simulink library "motohawk_control_primitives_motoshare_lib"  (Simulink 6.3)
undefined symbols (not defined in the file or in its folder): motohawk_vardec_config_group, motohawk_vardec_path, p, samp_time, SampleTime
libraries: MotoHawk_lib x76, motohawk_control_primitives_lib x30, simulink x9
(part 2 of 3)

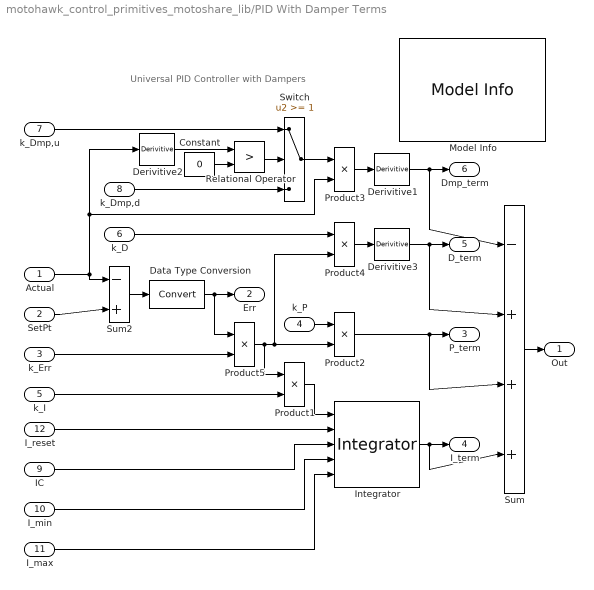
== system motohawk_control_primitives_motoshare_lib/PID With Damper Terms ==
  note: Universal PID Controller
      | with Dampers
  Actual : Inport
  SetPt : Inport  Port=2
  k_Err : Inport  Port=3
  k_P : Inport  Port=4
  k_I : Inport  Port=5
  k_D : Inport  Port=6
  k_Dmp,u : Inport  Port=7
  k_Dmp,d : Inport  Port=8
  IC : Inport  Port=9
  I_min : Inport  Port=10
  I_max : Inport  Port=11
  I_reset : Inport  Port=12
  Constant : Constant  Value=0
  Data Type Conversion : DataTypeConversion  SaturateOnIntegerOverflow=on  RndMeth=Zero
  Derivitive1 : motohawk_control_primitives_lib/Derivitive  samp_time=samp_time
  Derivitive2 : motohawk_control_primitives_lib/Derivitive  samp_time=samp_time
  Derivitive3 : motohawk_control_primitives_lib/Derivitive  samp_time=samp_time
  Integrator : motohawk_control_primitives_lib/Integrator  samp_time=samp_time
  Model Info : simulink/Model-Wide Utilities/Model Info  InitialBlockCM=None  BlockCM=None  Frame=on  DisplayStringWithTags=|  HorizontalTextAlignment=Center  LeftAlignmentValue=0.5  SourceBlockDiagram=motohawk_control_primitives_lib  TagMaxNumber=20
      | Model Info:
      | Author: Suhre, Poorman
      | %<Created>
      | %<ModifiedDate>
      | Version: %<ModelVersion>
      | MotoTron Confidential
      | and Propietary
  Product{1..5} (5 alike) : Product  InputSameDT=on
  Relational Operator : RelationalOperator  Operator=>  ZeroCross=off  InputSameDT=on
  Sum : Sum  Inputs=-|+|+|+  SaturateOnIntegerOverflow=on  InputSameDT=on
  Sum2 : Sum  Inputs=-|+  SaturateOnIntegerOverflow=on  InputSameDT=on
  Switch : Switch  Threshold=1  ZeroCross=off  InputSameDT=on
  Out : Outport
  Err : Outport  Port=2
  P_term : Outport  Port=3
  I_term : Outport  Port=4
  D_term : Outport  Port=5
  Dmp_term : Outport  Port=6
  wires:
  Product3/1 -> Derivitive1/1
  k_Dmp,u/1 -> Switch/1
  k_Dmp,d/1 -> Switch/3
  Switch/1 -> Product3/1
  Derivitive2/1 -> Relational Operator/1
  Relational Operator/1 -> Switch/2
  Constant/1 -> Relational Operator/2
  I_max/1 -> Integrator/5
  I_min/1 -> Integrator/4
  Data Type Conversion/1 -> Product5/1, Err/1
  k_Err/1 -> Product5/2
  I_reset/1 -> Integrator/2
  Actual/1 -> Sum2/1, Derivitive2/1, Product3/2
  k_P/1 -> Product2/1
  k_I/1 -> Product1/2
  Product1/1 -> Integrator/1
  Product2/1 -> P_term/1, Sum/3
  Integrator/1 -> I_term/1, Sum/4
  Sum/1 -> Out/1
  IC/1 -> Integrator/3
  Product5/1 -> Product1/1, Product2/2, Product4/2
  Sum2/1 -> Data Type Conversion/1
  SetPt/1 -> Sum2/2
  k_D/1 -> Product4/1
  Product4/1 -> Derivitive3/1
  Derivitive3/1 -> D_term/1, Sum/2
  Derivitive1/1 -> Dmp_term/1, Sum/1

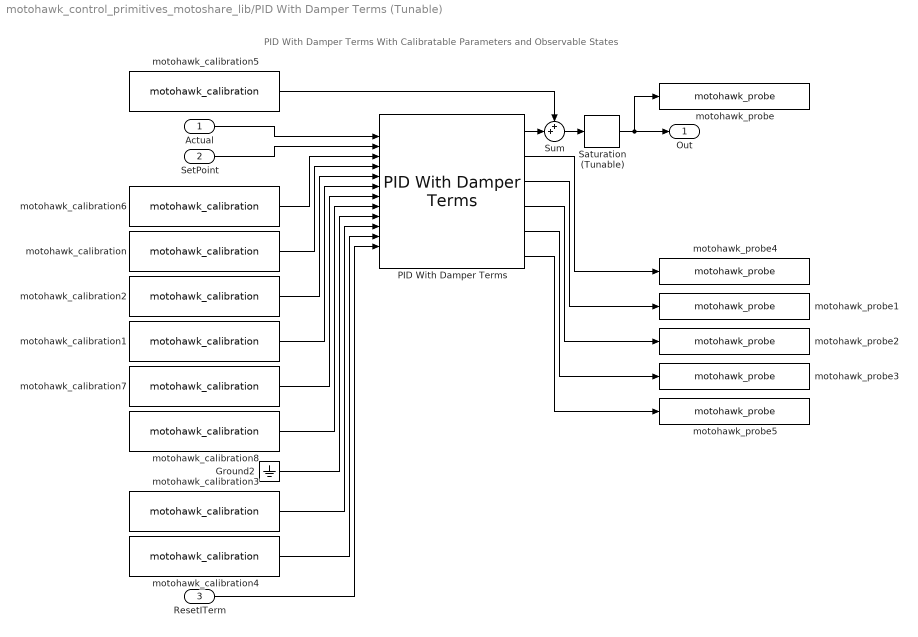
== system motohawk_control_primitives_motoshare_lib/PID With Damper Terms (Tunable) ==
  note: PID With Damper Terms
      | With Calibratable Parameters and Observable States
  Actual : Inport
  SetPoint : Inport  Port=2
  ResetITerm : Inport  Port=3
  Ground2 : Ground
  PID With Damper Terms : motohawk_control_primitives_lib/PID With Damper Terms  Description=|  samp_time=SampleTime
      | /* Name: ErrorGain Unit:mult ClassID:VAR StorageID:FLASH Access:RW4+RW3+NA2+NA1 TypeID:UINT4                   
      |    Gain:0.000000001 Min:0.000000000 Max:4.000000000 Format:10.9 UpdateID:REMOTE Help:"This gain is applied to "
      |    "the error term before it is used to calculate the P, I and D terms." VardecSig:6C */                       
      |                                                                                                                
      | /* Name: ITermLowerLim Unit:0 ClassID:VAR StorageID:FLASH Access:RW4+RW3+NA2+NA1 TypeID:SINT2 Gain:0.1         
      |    Min:-3276.8 Max:3276.7 Format:5.1 UpdateID:REMOTE Help:"Lower limit on the I-term value." VardecSig:6C */   
      |                                                                                                                
      | /* Name: ITermUpperLim ClassID:VAR StorageID:FLASH Access:RW4+RW3+NA2+NA1 TypeID:SINT2 Gain:0.1 Min:-3276.8    
      |    Max:3276.7 Format:5.1 UpdateID:REMOTE Help:"Upper limit on I-term value." VardecSig:6C */                   
      |                                                                                                                
      | /* Name: PIDOutLowerLim ClassID:VAR StorageID:FLASH Access:RW4+RW3+NA2+NA1 TypeID:SINT2 Gain:0.1               
      |    Min:-3276.8 Max:3276.7 Format:5.1 UpdateID:REMOTE Help:"Lower limit on PID output." VardecSig:6C */         
      |                                                                                                                
      | /* Name: PIDOutUpperLim ClassID:VAR StorageID:FLASH Access:RW4+RW3+NA2+NA1 TypeID:SINT2 Gain:0.1               
      |    Min:-3276.8 Max:3276.7 Format:3.1 UpdateID:REMOTE Help:"Upper limit on PID output." VardecSig:6C */         
      |                                                                                                                
      | /* Name: PIDError ClassID:VAR StorageID:RAM Access:RO4+RO3+NA2+NA1 TypeID:SINT2 Gain:1 Min:-32768.00           
      |    Max:32767.00 Format:4.2 UpdateID:BACKGND Help:"Current controller error input value." VardecSig:6C */       
      |                                                                                                                
      | /* Name: PTerm ClassID:VAR StorageID:RAM Access:RO4+RO3+NA2+NA1 TypeID:SINT2 Gain:1 Min:-32768.00              
      |    Max:32767.00 Format:4.2 UpdateID:BACKGND Help:"Current P-term value" VardecSig:6C */                        
      |                                                                                                                
      | /* Name: ITerm ClassID:VAR StorageID:RAM Access:RO4+RO3+NA2+NA1 TypeID:SINT2 Gain:1 Min:-32768.00              
      |    Max:32767.00 Format:4.2 UpdateID:BACKGND Help:"Current I-term value" VardecSig:6C */                        
      |                                                                                                                
      | /* Name: DTerm ClassID:VAR StorageID:RAM Access:RO4+RO3+NA2+NA1 TypeID:SINT2 Gain:1 Min:-32768.00              
      |    Max:32767.00 Format:4.2 UpdateID:BACKGND Help:"Current D-term value" VardecSig:6C */                        
      |                                                                                                                
      | /* Name: DamperTerm ClassID:VAR StorageID:RAM Access:RO4+RO3+NA2+NA1 TypeID:SINT2 Gain:1 Min:-32768.00         
      |    Max:32767.00 Format:4.2 UpdateID:BACKGND Help:"Current Damper-term value" VardecSig:6C */                   
      |                                                                                                                
      | /* Name: PIDOutput ClassID:VAR StorageID:FLASH Access:RW4+RW3+NA2+NA1 TypeID:SINT2 Gain:1 Min:-32768.00        
      |    Max:32767.00 Format:4.2 UpdateID:REMOTE Help:"PID current output." VardecSig:6C */
  Saturation (Tunable) : motohawk_control_primitives_lib/Saturation (Tunable)  prefix=prefix  units=units  grp=grp
  Sum : Sum  Inputs=++|  InputSameDT=on
  motohawk_calibration : MotoHawk_lib/Calibration & Probing Blocks/motohawk_calibration  nam=[prefix 'PGain']  val=1  storage=Calibration  show_more=on  name_source=Use Parameter  data_type=Inherit from 'Default Value'  read_level=1  write_level=1  ovr_cals=on  view_as=Number  enum_struct={'Disabled', 'Enabled'}  vector_style=Wide Row  use_help_units=on  help='PID Proportional Gain'  units='mult'  use_header_enum=off  row_header_enum={}  col_header_enum={}  use_min_max=off  min_val=-inf  max_val=inf  use_precision=off  precision=''  gain=1  offset=0  exp=1  use_mototune_group=on  mototune_group=grp
  motohawk_calibration1 : MotoHawk_lib/Calibration & Probing Blocks/motohawk_calibration  nam=[prefix 'DGain']  val=1  storage=Calibration  show_more=on  name_source=Use Parameter  data_type=Inherit from 'Default Value'  read_level=1  write_level=1  ovr_cals=on  view_as=Number  enum_struct={'Disabled', 'Enabled'}  vector_style=Wide Row  use_help_units=on  help='PID Derivative Gain'  units='mult'  use_header_enum=off  row_header_enum={}  col_header_enum={}  use_min_max=off  min_val=-inf  max_val=inf  use_precision=off  precision=''  gain=1  offset=0  exp=1  use_mototune_group=on  mototune_group=grp
  motohawk_calibration2 : MotoHawk_lib/Calibration & Probing Blocks/motohawk_calibration  nam=[prefix 'IGain']  val=1  storage=Calibration  show_more=on  name_source=Use Parameter  data_type=Inherit from 'Default Value'  read_level=1  write_level=1  ovr_cals=on  view_as=Number  enum_struct={'Disabled', 'Enabled'}  vector_style=Wide Row  use_help_units=on  help='PID Integral Gain'  units='mult'  use_header_enum=off  row_header_enum={}  col_header_enum={}  use_min_max=off  min_val=-inf  max_val=inf  use_precision=off  precision=''  gain=1  offset=0  exp=1  use_mototune_group=on  mototune_group=grp
  motohawk_calibration3 : MotoHawk_lib/Calibration & Probing Blocks/motohawk_calibration  nam=[prefix 'IMin']  val=0  storage=Calibration  show_more=on  name_source=Use Parameter  data_type=Inherit from 'Default Value'  read_level=1  write_level=1  ovr_cals=on  view_as=Number  enum_struct={'Disabled', 'Enabled'}  vector_style=Wide Row  use_help_units=on  help='PID Integrator Lower Limit'  units=units  use_header_enum=off  row_header_enum={}  col_header_enum={}  use_min_max=off  min_val=-inf  max_val=inf  use_precision=off  precision=''  gain=1  offset=0  exp=1  use_mototune_group=on  mototune_group=grp
  motohawk_calibration4 : MotoHawk_lib/Calibration & Probing Blocks/motohawk_calibration  nam=[prefix 'IMax']  val=1  storage=Calibration  show_more=on  name_source=Use Parameter  data_type=Inherit from 'Default Value'  read_level=1  write_level=1  ovr_cals=on  view_as=Number  enum_struct={'Disabled', 'Enabled'}  vector_style=Wide Row  use_help_units=on  help='PID Integrator Upper Limit'  units=units  use_header_enum=off  row_header_enum={}  col_header_enum={}  use_min_max=off  min_val=-inf  max_val=inf  use_precision=off  precision=''  gain=1  offset=0  exp=1  use_mototune_group=on  mototune_group=grp
  motohawk_calibration5 : MotoHawk_lib/Calibration & Probing Blocks/motohawk_calibration  nam=[prefix 'DCOffset']  val=0  storage=Calibration  show_more=on  name_source=Use Parameter  data_type=Inherit from 'Default Value'  read_level=1  write_level=1  ovr_cals=on  view_as=Number  enum_struct={'Disabled', 'Enabled'}  vector_style=Wide Row  use_help_units=on  help='PID Output DC Offset'  units=units  use_header_enum=off  row_header_enum={}  col_header_enum={}  use_min_max=off  min_val=-inf  max_val=inf  use_precision=off  precision=''  gain=1  offset=0  exp=1  use_mototune_group=on  mototune_group=grp
  motohawk_calibration6 : MotoHawk_lib/Calibration & Probing Blocks/motohawk_calibration  nam=[prefix 'ErrorGain']  val=1  storage=Calibration  show_more=on  name_source=Use Parameter  data_type=Inherit from 'Default Value'  read_level=1  write_level=1  ovr_cals=on  view_as=Number  enum_struct={'Disabled', 'Enabled'}  vector_style=Wide Row  use_help_units=on  help='PID Error Gain'  units='mult'  use_header_enum=off  row_header_enum={}  col_header_enum={}  use_min_max=off  min_val=-inf  max_val=inf  use_precision=off  precision=''  gain=1  offset=0  exp=1  use_mototune_group=on  mototune_group=grp
  motohawk_calibration7 : MotoHawk_lib/Calibration & Probing Blocks/motohawk_calibration  nam=[prefix 'DampGainUp']  val=1  storage=Calibration  show_more=on  name_source=Use Parameter  data_type=Inherit from 'Default Value'  read_level=1  write_level=1  ovr_cals=on  view_as=Number  enum_struct={'Disabled', 'Enabled'}  vector_style=Wide Row  use_help_units=on  help='PID Damper Gain - Up Direction'  units='mult'  use_header_enum=off  row_header_enum={}  col_header_enum={}  use_min_max=off  min_val=-inf  max_val=inf  use_precision=off  precision=''  gain=1  offset=0  exp=1  use_mototune_group=on  mototune_group=grp
  motohawk_calibration8 : MotoHawk_lib/Calibration & Probing Blocks/motohawk_calibration  nam=[prefix 'DampGainDown']  val=1  storage=Calibration  show_more=on  name_source=Use Parameter  data_type=Inherit from 'Default Value'  read_level=1  write_level=1  ovr_cals=on  view_as=Number  enum_struct={'Disabled', 'Enabled'}  vector_style=Wide Row  use_help_units=on  help='PID Damper Gain - Down Direction'  units='mult'  use_header_enum=off  row_header_enum={}  col_header_enum={}  use_min_max=off  min_val=-inf  max_val=inf  use_precision=off  precision=''  gain=1  offset=0  exp=1  use_mototune_group=on  mototune_group=grp
  motohawk_probe : MotoHawk_lib/Calibration & Probing Blocks/motohawk_probe  nam=[prefix 'Out']  show_more=on  name_source=Use Parameter  read_level=1  view_as=Number  enum_struct={'Disabled', 'Enabled'}  vector_style=Wide Row  use_help_units=on  help='PID Final Output'  units=units  use_header_enum=off  row_header_enum={}  col_header_enum={}  use_precision=off  precision=''  gain=1  offset=0  exp=1  use_mototune_group=on  mototune_group=grp
  motohawk_probe1 : MotoHawk_lib/Calibration & Probing Blocks/motohawk_probe  nam=[prefix 'PTerm']  show_more=on  name_source=Use Parameter  read_level=1  view_as=Number  enum_struct={'Disabled', 'Enabled'}  vector_style=Wide Row  use_help_units=on  help='PID Proportional Term'  units=units  use_header_enum=off  row_header_enum={}  col_header_enum={}  use_precision=off  precision=''  gain=1  offset=0  exp=1  use_mototune_group=on  mototune_group=grp
  motohawk_probe2 : MotoHawk_lib/Calibration & Probing Blocks/motohawk_probe  nam=[prefix 'ITerm']  show_more=on  name_source=Use Parameter  read_level=1  view_as=Number  enum_struct={'Disabled', 'Enabled'}  vector_style=Wide Row  use_help_units=on  help='PID Integrator Term'  units=units  use_header_enum=off  row_header_enum={}  col_header_enum={}  use_precision=off  precision=''  gain=1  offset=0  exp=1  use_mototune_group=on  mototune_group=grp
  motohawk_probe3 : MotoHawk_lib/Calibration & Probing Blocks/motohawk_probe  nam=[prefix 'DTerm']  show_more=on  name_source=Use Parameter  read_level=1  view_as=Number  enum_struct={'Disabled', 'Enabled'}  vector_style=Wide Row  use_help_units=on  help='PID Derivative Term'  units=units  use_header_enum=off  row_header_enum={}  col_header_enum={}  use_precision=off  precision=''  gain=1  offset=0  exp=1  use_mototune_group=on  mototune_group=grp
  motohawk_probe4 : MotoHawk_lib/Calibration & Probing Blocks/motohawk_probe  nam=[prefix 'Error']  show_more=on  name_source=Use Parameter  read_level=1  view_as=Number  enum_struct={'Disabled', 'Enabled'}  vector_style=Wide Row  use_help_units=on  help='PID Error Term'  units=units  use_header_enum=off  row_header_enum={}  col_header_enum={}  use_precision=off  precision=''  gain=1  offset=0  exp=1  use_mototune_group=on  mototune_group=grp
  motohawk_probe5 : MotoHawk_lib/Calibration & Probing Blocks/motohawk_probe  nam=[prefix 'DampTerm']  show_more=on  name_source=Use Parameter  read_level=1  view_as=Number  enum_struct={'Disabled', 'Enabled'}  vector_style=Wide Row  use_help_units=on  help='PID Damper Term'  units=units  use_header_enum=off  row_header_enum={}  col_header_enum={}  use_precision=off  precision=''  gain=1  offset=0  exp=1  use_mototune_group=on  mototune_group=grp
  Out : Outport
  wires:
  motohawk_calibration5/1 -> Sum/1
  Sum/1 -> Saturation (Tunable)/1
  ResetITerm/1 -> PID With Damper Terms/12
  Ground2/1 -> PID With Damper Terms/9
  motohawk_calibration1/1 -> PID With Damper Terms/6
  motohawk_calibration2/1 -> PID With Damper Terms/5
  motohawk_calibration/1 -> PID With Damper Terms/4
  PID With Damper Terms/3 -> motohawk_probe1/1
  Actual/1 -> PID With Damper Terms/1
  SetPoint/1 -> PID With Damper Terms/2
  PID With Damper Terms/1 -> Sum/2
  motohawk_calibration6/1 -> PID With Damper Terms/3
  motohawk_calibration3/1 -> PID With Damper Terms/10
  motohawk_calibration4/1 -> PID With Damper Terms/11
  PID With Damper Terms/4 -> motohawk_probe2/1
  PID With Damper Terms/5 -> motohawk_probe3/1
  PID With Damper Terms/2 -> motohawk_probe4/1
  motohawk_calibration7/1 -> PID With Damper Terms/7
  motohawk_calibration8/1 -> PID With Damper Terms/8
  PID With Damper Terms/6 -> motohawk_probe5/1
  Saturation (Tunable)/1 -> Out/1, motohawk_probe/1

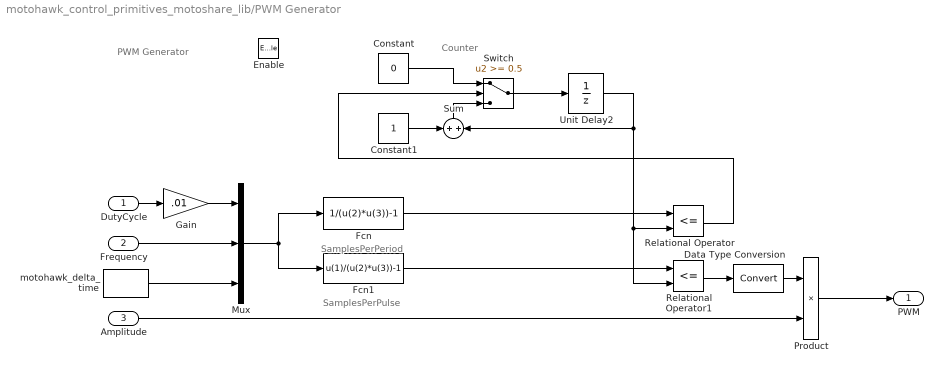
== system motohawk_control_primitives_motoshare_lib/PWM Generator ==
  note: Counter
  note: PWM Generator
  note: SamplesPerPulse
  note: SamplesPerPeriod
  DutyCycle : Inport
  Frequency : Inport  Port=2
  Amplitude : Inport  Port=3
  Enable : EnablePort  StatesWhenEnabling=reset
  Constant : Constant  Value=0
  Constant1 : Constant
  Data Type Conversion : DataTypeConversion  OutDataTypeMode=double  SaturateOnIntegerOverflow=on  RndMeth=Zero
  Fcn : Fcn  Expr=1/(u(2)*u(3))-1
  Fcn1 : Fcn  Expr=u(1)/(u(2)*u(3))-1
  Gain : Gain  Gain=.01  SaturateOnIntegerOverflow=on
  Mux : Mux  Inputs=3
  Product : Product  SaturateOnIntegerOverflow=on
  Relational Operator : RelationalOperator  Operator=<=
  Relational Operator1 : RelationalOperator  Operator=<=
  Sum : Sum  Orientation=up  SaturateOnIntegerOverflow=on  InputSameDT=on
  Switch : Switch  Threshold=0.5  SaturateOnIntegerOverflow=on  InputSameDT=on
  Unit Delay2 : UnitDelay  SampleTime=-1
  motohawk_delta_time : MotoHawk_lib/Extra Development Blocks/motohawk_delta_time  samp_time=-1  init_val=.005
  PWM : Outport  OutputWhenDisabled=reset  InitialOutput=0
  wires:
  Relational Operator/1 -> Switch/2
  Constant1/1 -> Sum/1
  Gain/1 -> Mux/1
  Data Type Conversion/1 -> Product/1
  Unit Delay2/1 -> Relational Operator1/2, Relational Operator/2, Sum/2
  Switch/1 -> Unit Delay2/1
  Constant/1 -> Switch/1
  Sum/1 -> Switch/3
  Amplitude/1 -> Product/2
  Product/1 -> PWM/1
  Relational Operator1/1 -> Data Type Conversion/1
  Fcn1/1 -> Relational Operator1/1
  Fcn/1 -> Relational Operator/1
  Mux/1 -> Fcn1/1, Fcn/1
  motohawk_delta_time/1 -> Mux/3
  Frequency/1 -> Mux/2
  DutyCycle/1 -> Gain/1

== system motohawk_control_primitives_motoshare_lib/Polynomial (Tunable) ==
  note: Evaluate polynomial using Horner's Rule.
      |      y = polyval( p, u, [], mu )
      | where
      |      p = polynomial coefficients and
      |      mu(1) = mean and
      |      mu(2) = standard deviation of fitted data.
      | See MATLAB "help polyfit" for more.
      | Note:  Degree of polynomial is fixed at compile time.
      | MotoTune can change coefficients, centering/scaling values.
  note: Evaluate Polynomial using Horner's Rule.
  u : Inport
  Constant : Constant  Value=[0 1]
  Demux : Demux  Outputs=2
  Horner's Rule : Subsystem
  Product0 : Product  Inputs=*/  SaturateOnIntegerOverflow=on
  Signal Specification0 : SignalSpecification  Dimensions=2
  Signal Specification1 : SignalSpecification  Dimensions=length(p)
  Sum : Sum  Inputs=|+-  SaturateOnIntegerOverflow=on  InputSameDT=on
  motohawk_calibration1 : MotoHawk_lib/Calibration & Probing Blocks/motohawk_calibration  nam=[prefix 'Polynomial']  val=ones(1,numcoef)  storage=Calibration  show_more=on  name_source=Use Parameter  data_type=Inherit from 'Default Value'  read_level=1  write_level=1  ovr_cals=on  view_as=Number  enum_struct={'Disabled', 'Enabled'}  vector_style=Wide Row  use_help_units=on  help='[ A_n ... A_0 ]'  units=''  use_header_enum=off  row_header_enum={}  col_header_enum={}  use_min_max=on  min_val=-inf  max_val=inf  use_precision=on  precision='1.14'  gain=1  offset=0  exp=1  use_mototune_group=on  mototune_group=grp
  y : Outport
  wires:
  Signal Specification0/1 -> Demux/1
  Signal Specification1/1 -> Horner's Rule/2(p)
  Horner's Rule/1(y) -> y/1
  motohawk_calibration1/1 -> Signal Specification1/1
  Product0/1 -> Horner's Rule/1(u_hat)
  Demux/2 -> Product0/2
  Constant/1 -> Signal Specification0/1
  Sum/1 -> Product0/1
  Demux/1 -> Sum/2
  u/1 -> Sum/1

== system motohawk_control_primitives_motoshare_lib/Rising Edge ==
  note: Detect Rising Edge of Signal
      | using Discrete Unit Delay
  In : Inport
  Data Type Conversion : DataTypeConversion  OutDataTypeMode=boolean  SaturateOnIntegerOverflow=on  RndMeth=Zero
  Logical Operator : Logic
  Logical Operator1 : Logic  Operator=NOT
  Unit Delay : UnitDelay  SampleTime=-1
  Rise : Outport
  wires:
  Data Type Conversion/1 -> Unit Delay/1, Logical Operator/1
  Logical Operator1/1 -> Logical Operator/2
  Unit Delay/1 -> Logical Operator1/1
  Logical Operator/1 -> Rise/1
  In/1 -> Data Type Conversion/1

== system motohawk_control_primitives_motoshare_lib/Saturate Divide ==
  note: When the divisor is less than the numerator,
      | saturate and output one.
  note: This is useful when dividing dT by a Time Constant.
      | It also avoids a divide by zero.
  X : Inport
  Inport : Inport  Port=2
  If : If  NumInputs=2  IfExpression=u2 < u1
  Merge : Merge
  Normal Divide : Subsystem
  Output One : Subsystem
  " " : Outport
  wires:
  X/1 -> Normal Divide/1(X), If/1
  Merge/1 -> " "/1
  Normal Divide/1(" ") -> Merge/1
  Output One/1(" ") -> Merge/2
  If/2 -> Normal Divide/Action
  If/1 -> Output One/Action
  Inport/1 -> Normal Divide/2(Inport), If/2

== system motohawk_control_primitives_motoshare_lib/Saturation ==
  note: Output 'In' when between Min and Max,
      | and saturate against limits otherwise.
  in : Inport
  min : Inport  Port=2
  max : Inport  Port=3
  MinMax : MinMax  Function=max  Inputs=2  ZeroCross=off  SaturateOnIntegerOverflow=on  InputSameDT=on
  MinMax1 : MinMax  Inputs=2  ZeroCross=off  SaturateOnIntegerOverflow=on  InputSameDT=on
  out : Outport
  wires:
  MinMax/1 -> MinMax1/1
  in/1 -> MinMax/1
  min/1 -> MinMax/2
  max/1 -> MinMax1/2
  MinMax1/1 -> out/1

== system motohawk_control_primitives_motoshare_lib/Saturation (Tunable) ==
  note: Calibratable wrapper around the Saturation block
  In : Inport
  Saturation : motohawk_control_primitives_lib/Saturation
  motohawk_calibration : MotoHawk_lib/Calibration & Probing Blocks/motohawk_calibration  nam=[prefix 'LwrLim']  val=0  storage=Calibration  show_more=on  name_source=Use Parameter  data_type=Inherit via back propagation  read_level=1  write_level=1  ovr_cals=on  view_as=Number  enum_struct={'Disabled', 'Enabled'}  vector_style=Wide Row  use_help_units=off  help='Lower Limit Value'  units=units  use_header_enum=off  row_header_enum={}  col_header_enum={}  use_min_max=on  min_val=-inf  max_val=inf  use_precision=off  precision=''  gain=1  offset=0  exp=1  use_mototune_group=on  mototune_group=grp
  motohawk_calibration1 : MotoHawk_lib/Calibration & Probing Blocks/motohawk_calibration  nam=[prefix 'UprLim']  val=1  storage=Calibration  show_more=on  name_source=Use Parameter  data_type=Inherit via back propagation  read_level=1  write_level=1  ovr_cals=on  view_as=Number  enum_struct={'Disabled', 'Enabled'}  vector_style=Wide Row  use_help_units=off  help='Upper Limit Value'  units=units  use_header_enum=off  row_header_enum={}  col_header_enum={}  use_min_max=on  min_val=-inf  max_val=inf  use_precision=off  precision=''  gain=1  offset=0  exp=1  use_mototune_group=on  mototune_group=grp
  Out : Outport
  wires:
  Saturation/1 -> Out/1
  motohawk_calibration/1 -> Saturation/2
  In/1 -> Saturation/1
  motohawk_calibration1/1 -> Saturation/3

== system motohawk_control_primitives_motoshare_lib/Simple PD ==
  note: Simple PD Controller
  Actual : Inport
  SetPt : Inport  Port=2
  k_P : Inport  Port=3
  k_D : Inport  Port=4
  Data Type Conversion1 : DataTypeConversion  SaturateOnIntegerOverflow=on  RndMeth=Zero
  Derivitive3 : motohawk_control_primitives_lib/Derivitive  samp_time=samp_time
  Model Info : simulink/Model-Wide Utilities/Model Info  InitialBlockCM=None  BlockCM=None  Frame=on  DisplayStringWithTags=|  HorizontalTextAlignment=Center  LeftAlignmentValue=0.5  SourceBlockDiagram=motohawk_control_primitives_lib  TagMaxNumber=20
      | Model Info:
      | Author: Poorman
      | %<ModifiedDate>
      | Version: %<ModelVersion>
      | MotoTron Confidential
      | and Propietary
  Product1 : Product  InputSameDT=on
  Product5 : Product  InputSameDT=on
  Sum1 : Sum  Inputs=+|+  SaturateOnIntegerOverflow=on  InputSameDT=on
  Sum2 : Sum  Inputs=-|||+  SaturateOnIntegerOverflow=on  InputSameDT=on
  Out : Outport
  wires:
  Data Type Conversion1/1 -> Product5/2, Product1/1
  Actual/1 -> Sum2/1
  k_P/1 -> Product1/2
  Sum2/1 -> Data Type Conversion1/1
  SetPt/1 -> Sum2/2
  k_D/1 -> Product5/1
  Product5/1 -> Derivitive3/1
  Sum1/1 -> Out/1
  Derivitive3/1 -> Sum1/1
  Product1/1 -> Sum1/2

== system motohawk_control_primitives_motoshare_lib/Simple PI ==
  note: Simple PI Controller
  Actual : Inport
  SetPt : Inport  Port=2
  k_P : Inport  Port=3
  k_I : Inport  Port=4
  Constant : Constant
  Constant1 : Constant  Value=-inf
  Constant2 : Constant  Value=inf
  Constant3 : Constant  Value=0
  Constant4 : Constant  Value=0
  Data Type Conversion : DataTypeConversion  SaturateOnIntegerOverflow=on  RndMeth=Zero
  Integrator : motohawk_control_primitives_lib/Integrator  samp_time=samp_time
  Model Info : simulink/Model-Wide Utilities/Model Info  InitialBlockCM=None  BlockCM=None  Frame=on  DisplayStringWithTags=|  HorizontalTextAlignment=Center  LeftAlignmentValue=0.5  SourceBlockDiagram=motohawk_control_primitives_lib  TagMaxNumber=20
      | Model Info:
      | Author: Poorman
      | %<Created>
      | %<ModifiedDate>
      | Version: %<ModelVersion>
      | MotoTron Confidential
      | and Propietary
  Product1 : Product  InputSameDT=on
  Product2 : Product  InputSameDT=on
  Product3 : Product  InputSameDT=on
  Sum : Sum  Inputs=+|+  SaturateOnIntegerOverflow=on  InputSameDT=on
  Sum2 : Sum  Inputs=-|+  SaturateOnIntegerOverflow=on  InputSameDT=on
  Out : Outport
  wires:
  Constant2/1 -> Integrator/5
  Constant1/1 -> Integrator/4
  Data Type Conversion/1 -> Product3/1
  Constant/1 -> Product3/2
  Constant4/1 -> Integrator/2
  SetPt/1 -> Sum2/2
  Actual/1 -> Sum2/1
  k_P/1 -> Product2/1
  k_I/1 -> Product1/2
  Product1/1 -> Integrator/1
  Product2/1 -> Sum/1
  Integrator/1 -> Sum/2
  Sum/1 -> Out/1
  Constant3/1 -> Integrator/3
  Product3/1 -> Product2/2, Product1/1
  Sum2/1 -> Data Type Conversion/1

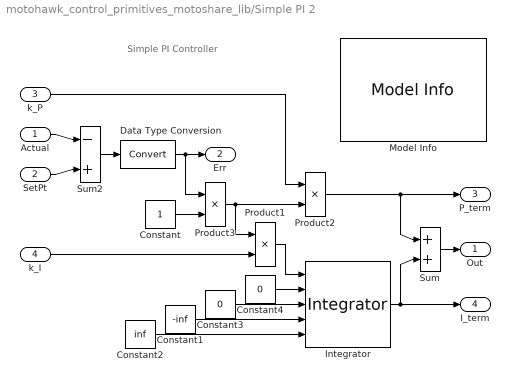
== system motohawk_control_primitives_motoshare_lib/Simple PI 2 ==
  note: Simple PI Controller
  Actual : Inport
  SetPt : Inport  Port=2
  k_P : Inport  Port=3
  k_I : Inport  Port=4
  Constant : Constant
  Constant1 : Constant  Value=-inf
  Constant2 : Constant  Value=inf
  Constant3 : Constant  Value=0
  Constant4 : Constant  Value=0
  Data Type Conversion : DataTypeConversion  SaturateOnIntegerOverflow=on  RndMeth=Zero
  Integrator : motohawk_control_primitives_lib/Integrator  samp_time=samp_time
  Model Info : simulink/Model-Wide Utilities/Model Info  InitialBlockCM=None  BlockCM=None  Frame=on  DisplayStringWithTags=|  HorizontalTextAlignment=Center  LeftAlignmentValue=0.5  SourceBlockDiagram=motohawk_control_primitives_lib  TagMaxNumber=20
      | Model Info:
      | Author: Poorman
      | %<Created>
      | %<ModifiedDate>
      | Version: %<ModelVersion>
      | MotoTron Confidential
      | and Propietary
  Product1 : Product  InputSameDT=on
  Product2 : Product  InputSameDT=on
  Product3 : Product  InputSameDT=on
  Sum : Sum  Inputs=+|+  SaturateOnIntegerOverflow=on  InputSameDT=on
  Sum2 : Sum  Inputs=-|+  SaturateOnIntegerOverflow=on  InputSameDT=on
  Out : Outport
  Err : Outport  Port=2
  P_term : Outport  Port=3
  I_term : Outport  Port=4
  wires:
  Sum2/1 -> Data Type Conversion/1
  Product3/1 -> Product1/1, Product2/2
  Constant3/1 -> Integrator/3
  Sum/1 -> Out/1
  Integrator/1 -> Sum/2, I_term/1
  Product2/1 -> Sum/1, P_term/1
  Product1/1 -> Integrator/1
  k_I/1 -> Product1/2
  k_P/1 -> Product2/1
  Actual/1 -> Sum2/1
  SetPt/1 -> Sum2/2
  Constant4/1 -> Integrator/2
  Constant/1 -> Product3/2
  Data Type Conversion/1 -> Product3/1, Err/1
  Constant1/1 -> Integrator/4
  Constant2/1 -> Integrator/5

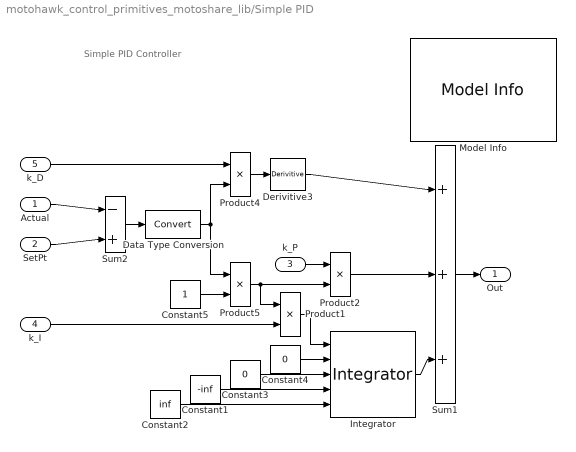
== system motohawk_control_primitives_motoshare_lib/Simple PID ==
  note: Simple PID Controller
  Actual : Inport
  SetPt : Inport  Port=2
  k_P : Inport  Port=3
  k_I : Inport  Port=4
  k_D : Inport  Port=5
  Constant1 : Constant  Value=-inf
  Constant2 : Constant  Value=inf
  Constant3 : Constant  Value=0
  Constant4 : Constant  Value=0
  Constant5 : Constant
  Data Type Conversion : DataTypeConversion  SaturateOnIntegerOverflow=on  RndMeth=Zero
  Derivitive3 : motohawk_control_primitives_lib/Derivitive  samp_time=samp_time
  Integrator : motohawk_control_primitives_lib/Integrator  samp_time=samp_time
  Model Info : simulink/Model-Wide Utilities/Model Info  InitialBlockCM=None  BlockCM=None  Frame=on  DisplayStringWithTags=|  HorizontalTextAlignment=Center  LeftAlignmentValue=0.5  SourceBlockDiagram=motohawk_control_primitives_lib  TagMaxNumber=20
      | Model Info:
      | Author: Suhre, Poorman
      | %<Created>
      | %<ModifiedDate>
      | Version: %<ModelVersion>
      | MotoTron Confidential
      | and Propietary
  Product{1..2,4..5} (4 alike) : Product  InputSameDT=on
  Sum1 : Sum  Inputs=+|+|+  SaturateOnIntegerOverflow=on  InputSameDT=on
  Sum2 : Sum  Inputs=-|+  SaturateOnIntegerOverflow=on  InputSameDT=on
  Out : Outport
  wires:
  Data Type Conversion/1 -> Product5/1, Product4/2
  Constant5/1 -> Product5/2
  Actual/1 -> Sum2/1
  k_P/1 -> Product2/1
  k_I/1 -> Product1/2
  Product1/1 -> Integrator/1
  Product2/1 -> Sum1/2
  Integrator/1 -> Sum1/3
  Sum1/1 -> Out/1
  Product5/1 -> Product2/2, Product1/1
  Sum2/1 -> Data Type Conversion/1
  SetPt/1 -> Sum2/2
  k_D/1 -> Product4/1
  Product4/1 -> Derivitive3/1
  Derivitive3/1 -> Sum1/1
  Constant2/1 -> Integrator/5
  Constant1/1 -> Integrator/4
  Constant3/1 -> Integrator/3
  Constant4/1 -> Integrator/2

== system motohawk_control_primitives_motoshare_lib/Switch Debounce ==
  SwIn : Inport
  Period [s] : Inport  Port=2
  Logical Operator : Logic  Operator=NOT  AllPortsSameDT=off  OutDataTypeMode=Boolean
  Relational Operator : RelationalOperator  LogicOutDataTypeMode=Boolean
  Relational Operator1 : RelationalOperator  LogicOutDataTypeMode=Boolean
  Switch Debounce State Machine : Stateflow chart  TreatAsAtomicUnit=on
  Time Since Enabled (With Input) : motohawk_control_primitives_lib/Time Since Enabled (With Input)  samp_time=-1  init=0
  Time Since Enabled (With Input)1 : motohawk_control_primitives_lib/Time Since Enabled (With Input)  samp_time=-1  init=0
  SwOut : Outport
  wires:
  Switch Debounce State Machine/1(State) -> SwOut/1
  Time Since Enabled (With Input)/1 -> Relational Operator/1
  Period [s]/1 -> Relational Operator/2, Relational Operator1/2
  SwIn/1 -> Time Since Enabled (With Input)/Enable, Switch Debounce State Machine/3(SwIn), Logical Operator/1
  Time Since Enabled (With Input)1/1 -> Relational Operator1/1
  Relational Operator/1 -> Switch Debounce State Machine/1(OffToOnTrsn)
  Relational Operator1/1 -> Switch Debounce State Machine/2(OnToOffTrsn)
  Logical Operator/1 -> Time Since Enabled (With Input)1/Enable

== system motohawk_control_primitives_motoshare_lib/Time Since Enabled ==
  note: Output the time since enabled, by summing up 'dt'.
  note: If this block is in an enabled subsystem that
      | resets its states, then the count will reset as well.
      | Otherwise, the count will resume from where it left off.
      |
      | Note that when the Sample Time of the the 'dt' is non-positive,
      | the block will only output its Initial Value if the enabled subsystem
      | is set to reset its state.  This means that the count will immediately
      | 'catch up' if the enabled subsystem holds its states.
  Sum : Sum  Inputs=|++  SaturateOnIntegerOverflow=on  InputSameDT=on
  Unit Delay : UnitDelay  SampleTime=-1
  motohawk_delta_time : MotoHawk_lib/Extra Development Blocks/motohawk_delta_time  samp_time=samp_time  init_val=0
  Time Since Enabled [sec] : Outport
  wires:
  Unit Delay/1 -> Time Since Enabled [sec]/1, Sum/2
  Sum/1 -> Unit Delay/1
  motohawk_delta_time/1 -> Sum/1

== system motohawk_control_primitives_motoshare_lib/Time Since Enabled (With Input) ==
  note: Output the time since enabled, by summing up 'dt'.
      | States are reset when re-enabled.
      | Output is reset to zero when disabled.
  Enable : EnablePort  StatesWhenEnabling=reset  ZeroCross=off
  Sum : Sum  Inputs=|++  SaturateOnIntegerOverflow=on  InputSameDT=on
  Unit Delay : UnitDelay  SampleTime=-1
  motohawk_delta_time : MotoHawk_lib/Extra Development Blocks/motohawk_delta_time  samp_time=samp_time  init_val=0
  Time Since Enabled [sec] : Outport  OutputWhenDisabled=reset  InitialOutput=init
  wires:
  motohawk_delta_time/1 -> Sum/1
  Sum/1 -> Unit Delay/1
  Unit Delay/1 -> Sum/2, Time Since Enabled [sec]/1

== system motohawk_control_primitives_motoshare_lib/Triggered Counter Falling ==
  note: Triggered Counter
  Reset : Inport
  Increment : Inport  Port=2
  Trigger : TriggerPort  TriggerType=falling
  Constant : Constant  Value=0
  Sum : Sum  Orientation=up  SaturateOnIntegerOverflow=on  InputSameDT=on
  Switch : Switch  Threshold=0.5  SaturateOnIntegerOverflow=on  InputSameDT=on
  Unit Delay1 : UnitDelay  Orientation=left  SampleTime=-1
  Counter : Outport
  wires:
  Unit Delay1/1 -> Sum/2
  Increment/1 -> Sum/1
  Reset/1 -> Switch/2
  Switch/1 -> Unit Delay1/1, Counter/1
  Constant/1 -> Switch/1
  Sum/1 -> Switch/3

== system motohawk_control_primitives_motoshare_lib/Triggered Counter Rising ==
  note: Triggered Counter
  Reset : Inport
  Increment : Inport  Port=2
  Trigger : TriggerPort
  Constant : Constant  Value=0
  Sum : Sum  Orientation=up  SaturateOnIntegerOverflow=on  InputSameDT=on
  Switch : Switch  Threshold=0.5  SaturateOnIntegerOverflow=on  InputSameDT=on
  Unit Delay1 : UnitDelay  Orientation=left  SampleTime=-1
  Counter : Outport
  wires:
  Switch/1 -> Counter/1, Unit Delay1/1
  Reset/1 -> Switch/2
  Constant/1 -> Switch/1
  Sum/1 -> Switch/3
  Increment/1 -> Sum/1
  Unit Delay1/1 -> Sum/2

== system motohawk_control_primitives_motoshare_lib/Universal PD ==
  note: Universal PD Controller
  Actual : Inport
  SetPt : Inport  Port=2
  k_Err : Inport  Port=3
  k_P : Inport  Port=4
  k_D : Inport  Port=5
  Data Type Conversion : DataTypeConversion  SaturateOnIntegerOverflow=on  RndMeth=Zero
  Derivitive : motohawk_control_primitives_lib/Derivitive  samp_time=samp_time
  Model Info : simulink/Model-Wide Utilities/Model Info  InitialBlockCM=None  BlockCM=None  Frame=on  DisplayStringWithTags=|  HorizontalTextAlignment=Center  LeftAlignmentValue=0.5  SourceBlockDiagram=motohawk_control_primitives_lib  TagMaxNumber=20
      | Model Info:
      | Author: %<Creator>
      | %<Created>
      | %<ModifiedDate>
      | Version: %<ModelVersion>
      | MotoTron Confidential
      | and Propietary
  Product : Product  InputSameDT=on
  Product2 : Product  InputSameDT=on
  Product4 : Product  InputSameDT=on
  Sum : Sum  SaturateOnIntegerOverflow=on  InputSameDT=on
  Sum1 : Sum  Inputs=|-+
  Out : Outport
  Err : Outport  Port=2
  P_term : Outport  Port=3
  D_term : Outport  Port=4
  wires:
  Product4/1 -> Product2/1, Product/1
  Sum/1 -> Out/1
  Derivitive/1 -> Sum/2, D_term/1
  Product/1 -> Sum/1, P_term/1
  Product2/1 -> Derivitive/1
  k_D/1 -> Product2/2
  k_P/1 -> Product/2
  Actual/1 -> Sum1/1
  SetPt/1 -> Sum1/2
  Sum1/1 -> Data Type Conversion/1
  k_Err/1 -> Product4/2
  Data Type Conversion/1 -> Product4/1, Err/1

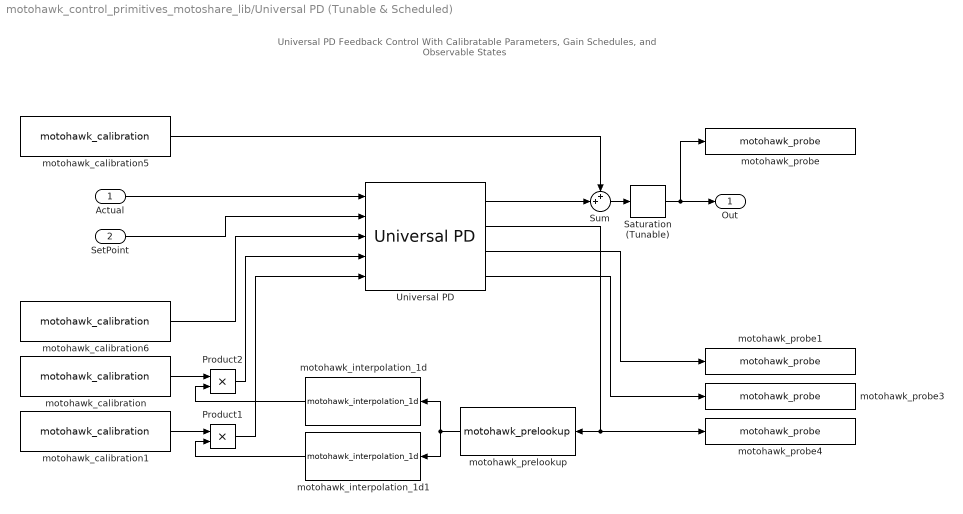
== system motohawk_control_primitives_motoshare_lib/Universal PD (Tunable & Scheduled) ==
  note: Universal PD Feedback Control
      | With Calibratable Parameters,
      | Gain Schedules, and Observable States
  Actual : Inport
  SetPoint : Inport  Port=2
  Product1 : Product  SaturateOnIntegerOverflow=on  InputSameDT=on
  Product2 : Product  SaturateOnIntegerOverflow=on  InputSameDT=on
  Saturation (Tunable) : motohawk_control_primitives_lib/Saturation (Tunable)  prefix=prefix  units=units  grp=motohawk_vardec_config_group(grp)
  Sum : Sum  Inputs=++|  InputSameDT=on
  Universal PD : motohawk_control_primitives_lib/Universal PD  Description=|  samp_time=SampleTime
      | /* Name: ErrorGain Unit:mult ClassID:VAR StorageID:FLASH Access:RW4+RW3+NA2+NA1 TypeID:UINT4                   
      |    Gain:0.000000001 Min:0.000000000 Max:4.000000000 Format:10.9 UpdateID:REMOTE Help:"This gain is applied to "
      |    "the error term before it is used to calculate the P, I and D terms." VardecSig:6C */                       
      |                                                                                                                
      | /* Name: ITermLowerLim Unit:0 ClassID:VAR StorageID:FLASH Access:RW4+RW3+NA2+NA1 TypeID:SINT2 Gain:0.1         
      |    Min:-3276.8 Max:3276.7 Format:5.1 UpdateID:REMOTE Help:"Lower limit on the I-term value." VardecSig:6C */   
      |                                                                                                                
      | /* Name: ITermUpperLim ClassID:VAR StorageID:FLASH Access:RW4+RW3+NA2+NA1 TypeID:SINT2 Gain:0.1 Min:-3276.8    
      |    Max:3276.7 Format:5.1 UpdateID:REMOTE Help:"Upper limit on I-term value." VardecSig:6C */                   
      |                                                                                                                
      | /* Name: PIDOutLowerLim ClassID:VAR StorageID:FLASH Access:RW4+RW3+NA2+NA1 TypeID:SINT2 Gain:0.1               
      |    Min:-3276.8 Max:3276.7 Format:5.1 UpdateID:REMOTE Help:"Lower limit on PID output." VardecSig:6C */         
      |                                                                                                                
      | /* Name: PIDOutUpperLim ClassID:VAR StorageID:FLASH Access:RW4+RW3+NA2+NA1 TypeID:SINT2 Gain:0.1               
      |    Min:-3276.8 Max:3276.7 Format:3.1 UpdateID:REMOTE Help:"Upper limit on PID output." VardecSig:6C */
  motohawk_calibration : MotoHawk_lib/Calibration & Probing Blocks/motohawk_calibration  nam=[prefix 'PGain']  val=1  storage=Calibration  show_more=on  name_source=Use Parameter  data_type=Inherit from 'Default Value'  read_level=1  write_level=1  ovr_cals=on  view_as=Number  enum_struct={'Disabled', 'Enabled'}  vector_style=Wide Row  use_help_units=on  help='PID Proportional Gain'  units='mult'  use_header_enum=off  row_header_enum={}  col_header_enum={}  use_min_max=off  min_val=-inf  max_val=inf  use_precision=off  precision=''  gain=1  offset=0  exp=1  use_mototune_group=on  mototune_group=motohawk_vardec_config_group(grp)
  motohawk_calibration1 : MotoHawk_lib/Calibration & Probing Blocks/motohawk_calibration  nam=[prefix 'DGain']  val=1  storage=Calibration  show_more=on  name_source=Use Parameter  data_type=Inherit from 'Default Value'  read_level=1  write_level=1  ovr_cals=on  view_as=Number  enum_struct={'Disabled', 'Enabled'}  vector_style=Wide Row  use_help_units=on  help='PID Derivative Gain'  units='mult'  use_header_enum=off  row_header_enum={}  col_header_enum={}  use_min_max=off  min_val=-inf  max_val=inf  use_precision=off  precision=''  gain=1  offset=0  exp=1  use_mototune_group=on  mototune_group=motohawk_vardec_config_group(grp)
  motohawk_calibration5 : MotoHawk_lib/Calibration & Probing Blocks/motohawk_calibration  nam=[prefix 'DCOffset']  val=0  storage=Calibration  show_more=on  name_source=Use Parameter  data_type=Inherit from 'Default Value'  read_level=1  write_level=1  ovr_cals=on  view_as=Number  enum_struct={'Disabled', 'Enabled'}  vector_style=Wide Row  use_help_units=on  help='PID Output DC Offset'  units=units  use_header_enum=off  row_header_enum={}  col_header_enum={}  use_min_max=off  min_val=-inf  max_val=inf  use_precision=off  precision=''  gain=1  offset=0  exp=1  use_mototune_group=on  mototune_group=motohawk_vardec_config_group(grp)
  motohawk_calibration6 : MotoHawk_lib/Calibration & Probing Blocks/motohawk_calibration  nam=[prefix 'ErrorGain']  val=1  storage=Calibration  show_more=on  name_source=Use Parameter  data_type=Inherit from 'Default Value'  read_level=1  write_level=1  ovr_cals=on  view_as=Number  enum_struct={'Disabled', 'Enabled'}  vector_style=Wide Row  use_help_units=on  help='PID Error Gain'  units='mult'  use_header_enum=off  row_header_enum={}  col_header_enum={}  use_min_max=off  min_val=-inf  max_val=inf  use_precision=off  precision=''  gain=1  offset=0  exp=1  use_mototune_group=on  mototune_group=motohawk_vardec_config_group(grp)
  motohawk_interpolation_1d : MotoHawk_lib/Lookup Tables/motohawk_interpolation_1d  Orientation=left  nam=[prefix 'PMult']  table_data=ones(1,tblsize)  show_more=on  data_type=Inherit from 'Table Data'  storage=NonAdaptive  read_level=1  write_level=1  ovr_cals=on  use_help=on  help='Proportional term gain schedule'  units='mult'  use_min_max=off  min_val=-inf  max_val=inf  use_precision=off  precision=''  gain=1  offset=0  exp=1  use_links=off  prelookup_block=''  output_name=''  use_mototune_group=on  mototune_group=grp
  motohawk_interpolation_1d1 : MotoHawk_lib/Lookup Tables/motohawk_interpolation_1d  Orientation=left  nam=[prefix 'DMult']  table_data=ones(1,tblsize)  show_more=on  data_type=Inherit from 'Table Data'  storage=NonAdaptive  read_level=1  write_level=1  ovr_cals=on  use_help=on  help='Derivative term gain schedule'  units='mult'  use_min_max=off  min_val=-inf  max_val=inf  use_precision=off  precision=''  gain=1  offset=0  exp=1  use_links=off  prelookup_block=''  output_name=''  use_mototune_group=on  mototune_group=grp
  motohawk_prelookup : MotoHawk_lib/Lookup Tables/motohawk_prelookup  Orientation=left  nam=[prefix 'Error']  breakpoint_data=ones(1,tblsize)  show_more=on  data_type=Inherit from 'Table Data'  storage=Constant  read_level=1  write_level=1  ovr_cals=on  use_help=on  help='Error gain schedule ordinates'  units=units  use_min_max=off  min_val=-inf  max_val=inf  use_precision=off  precision=''  gain=1  offset=0  exp=1  use_links=on  input_name=[prefix 'Error']  use_mototune_group=on  mototune_group=grp
  motohawk_probe : MotoHawk_lib/Calibration & Probing Blocks/motohawk_probe  nam=[prefix 'Out']  show_more=on  name_source=Use Parameter  read_level=1  view_as=Number  enum_struct={'Disabled', 'Enabled'}  vector_style=Wide Row  use_help_units=on  help='PID Final Output'  units=units  use_header_enum=off  row_header_enum={}  col_header_enum={}  use_precision=off  precision=''  gain=1  offset=0  exp=1  use_mototune_group=on  mototune_group=grp
  motohawk_probe1 : MotoHawk_lib/Calibration & Probing Blocks/motohawk_probe  nam=[prefix 'PTerm']  show_more=on  name_source=Use Parameter  read_level=1  view_as=Number  enum_struct={'Disabled', 'Enabled'}  vector_style=Wide Row  use_help_units=on  help='PID Proportional Term'  units=units  use_header_enum=off  row_header_enum={}  col_header_enum={}  use_precision=off  precision=''  gain=1  offset=0  exp=1  use_mototune_group=on  mototune_group=grp
  motohawk_probe3 : MotoHawk_lib/Calibration & Probing Blocks/motohawk_probe  nam=[prefix 'DTerm']  show_more=on  name_source=Use Parameter  read_level=1  view_as=Number  enum_struct={'Disabled', 'Enabled'}  vector_style=Wide Row  use_help_units=on  help='PID Derivative Term'  units=units  use_header_enum=off  row_header_enum={}  col_header_enum={}  use_precision=off  precision=''  gain=1  offset=0  exp=1  use_mototune_group=on  mototune_group=grp
  motohawk_probe4 : MotoHawk_lib/Calibration & Probing Blocks/motohawk_probe  nam=[prefix 'Error']  show_more=on  name_source=Use Parameter  read_level=1  view_as=Number  enum_struct={'Disabled', 'Enabled'}  vector_style=Wide Row  use_help_units=on  help='PID Error Term'  units=units  use_header_enum=off  row_header_enum={}  col_header_enum={}  use_precision=off  precision=''  gain=1  offset=0  exp=1  use_mototune_group=on  mototune_group=grp
  Out : Outport
  wires:
  motohawk_prelookup/1 -> motohawk_interpolation_1d1/1, motohawk_interpolation_1d/1
  SetPoint/1 -> Universal PD/2
  Actual/1 -> Universal PD/1
  Saturation (Tunable)/1 -> motohawk_probe/1, Out/1
  Universal PD/2 -> motohawk_prelookup/1, motohawk_probe4/1
  Universal PD/4 -> motohawk_probe3/1
  Universal PD/1 -> Sum/2
  Universal PD/3 -> motohawk_probe1/1
  Sum/1 -> Saturation (Tunable)/1
  motohawk_calibration5/1 -> Sum/1
  motohawk_calibration6/1 -> Universal PD/3
  Product2/1 -> Universal PD/4
  motohawk_calibration/1 -> Product2/1
  Product1/1 -> Universal PD/5
  motohawk_calibration1/1 -> Product1/1
  motohawk_interpolation_1d/1 -> Product2/2
  motohawk_interpolation_1d1/1 -> Product1/2
